simulink model "adcs_model"  (R2025a)
settings: Solver=VariableStepAuto  StartTime=0.0  StopTime=10.0  RelTol=1e-3
InitFcn:
  | init;
settings Model: Creator=arroy  LastModifiedBy=arroy

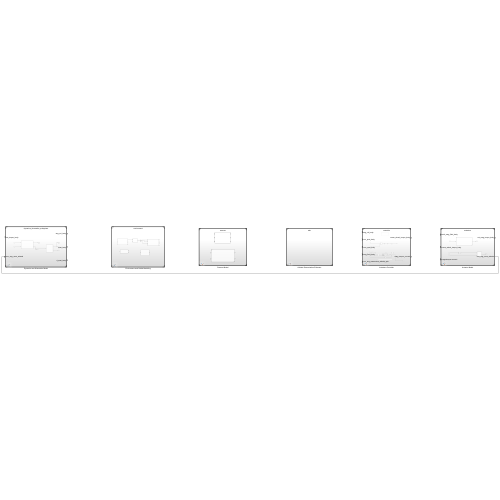
[thumbnail: Simulink's stored preview of the top-level diagram]
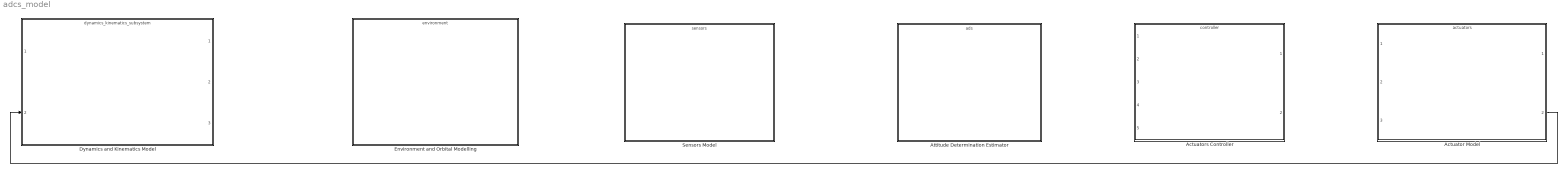
== system adcs_model ==
  Actuator Model : ModelReference  ModelNameDialog=actuators.slx  SimulationMode=Normal  ModelReferenceVersion=1.3
  Actuators Controller : ModelReference  ModelNameDialog=controller.slx  SimulationMode=Normal  ModelReferenceVersion=1.2
  Attitude Determination Estimator : ModelReference  ModelNameDialog=ads.slx  SimulationMode=Normal  ModelReferenceVersion=1.1
  Dynamics and Kinematics Model : ModelReference  ModelNameDialog=dynamics_kinematics_subsystem.slx  SimulationMode=Normal  ModelReferenceVersion=1.2
  Environment and Orbital Modelling : ModelReference  ModelNameDialog=environment.slx  SimulationMode=Normal  ModelReferenceVersion=1.4
  Sensors Model : ModelReference  ModelNameDialog=sensors.slx  SimulationMode=Normal  ModelReferenceVersion=1.1
  wires:
  Actuator Model/2 -> Dynamics and Kinematics Model/2
